simulink model "attitude_controllerV6"  (R2025a)
settings: Solver=FixedStepDiscrete  StartTime=0.0  StopTime=40  FixedStep=1e-4  RelTol=1e-6
undefined symbols (not defined in the file or in its folder): DiscIntNeverNeededParam
libraries: simulink x18, cstblocks x14, slpidlib x6, aerolibutil x2, rllib x1
(part 2 of 2)

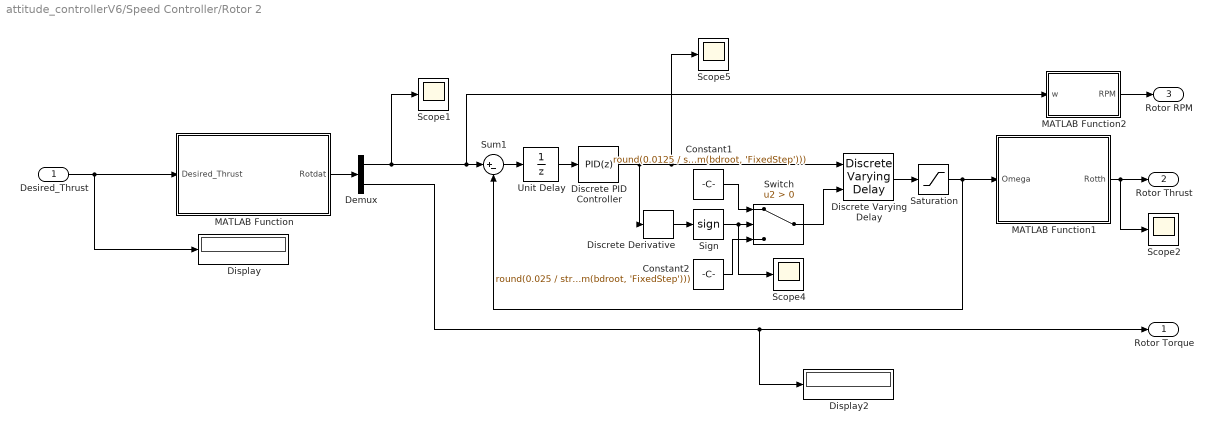
== system attitude_controllerV6/Speed Controller/Rotor 2 ==
  Desired_Thrust : Inport
  Constant1 : Constant  Value=round(0.0125 / str2double(get_param(bdroot, 'FixedStep')))
  Constant2 : Constant  Value=round(0.025 / str2double(get_param(bdroot, 'FixedStep')))
  Demux : Demux  Outputs=2
  Discrete Derivative : simulink/Discrete/Discrete Derivative  gainval=1.0  ICPrevScaledInput=0.0  OutMin=[]  OutMax=[]  OutDataType=fixdt(1, 16)  OutScaling=2^-10  DoSatur=off
  Discrete PID Controller : slpidlib/PID Controller  Controller=PID  Form=Parallel  TimeDomain=Discrete-time  UseExternalTs=off  SampleTime=-1  IntegratorMethod=Forward Euler  FilterMethod=Forward Euler  ControllerParametersSource=internal  P=0  I=30  UseKiTs=off  D=0  UseExternalDerivativeSource=off  N=100  UseFilter=on  TunerSelectOption=Transfer Function Based (PID Tuner App)  InitialConditionSource=internal  InitialConditionForIntegrator=0  InitialConditionForFilter=0  DifferentiatorICPrevScaledInput=0  ExternalReset=none  TrackingMode=off  Kt=1  LimitOutput=off  SatLimitsSource=internal  UpperSaturationLimit=inf  LowerSaturationLimit=-inf  LinearizeAsGain=off  AntiWindupMode=none  Kb=1  LimitIntegrator=off  UpperIntegratorSaturationLimit=inf  LowerIntegratorSaturationLimit=-inf  POutMin=[]  POutMax=[]  IOutMin=[]  IOutMax=[]  DOutMin=[]  DOutMax=[]  NOutMin=[]  NOutMax=[]  SumOutMin=[]  SumOutMax=[]  SaturationOutMin=[]  SaturationOutMax=[]  PParamMin=[]  PParamMax=[]  IParamMin=[]  IParamMax=[]  DParamMin=[]  DParamMax=[]  NParamMin=[]  NParamMax=[]  KbParamMin=[]  KbParamMax=[]  KtParamMin=[]  KtParamMax=[]  KbOutMin=[]  KbOutMax=[]  KtOutMin=[]  KtOutMax=[]  IntegratorOutMin=[]  IntegratorOutMax=[]  FilterOutMin=[]  FilterOutMax=[]  SumI1OutMin=[]  SumI1OutMax=[]  SumI2OutMin=[]  SumI2OutMax=[]  SumI3OutMin=[]  SumI3OutMax=[]  SumI4OutMin=[]  SumI4OutMax=[]  SumDOutMin=[]  SumDOutMax=[]  DifferentiatorOutMin=[]  DifferentiatorOutMax=[]  FilterDiffOutCoefMin=[]  FilterDiffOutCoefMax=[]  ReciprocalOutMin=[]  ReciprocalOutMax=[]  SumDenOutMin=[]  SumDenOutMax=[]  SumNumOutMin=[]  SumNumOutMax=[]  DivideOutMin=[]  DivideOutMax=[]  UdiffTsProdOutMin=[]  UdiffTsProdOutMax=[]  NTsProdOutMin=[]  NTsProdOutMax=[]  UintegralTsProdOutMin=[]  UintegralTsProdOutMax=[]  UngainTsProdOutMin=[]  UngainTsProdOutMax=[]  ClampingZeroOutDataTypeStr=Inherit: Inherit via back propagation  ClampingZeroOutMin=[]  ClampingZeroOutMax=[]  FilterDenConstantOutDataTypeStr=Inherit: Inherit via back propagation  FilterDenConstantOutMin=[]  FilterDenConstantOutMax=[]  PCopyOutDataTypeStr=Inherit: Inherit via back propagation  PCopyOutMin=[]  PCopyOutMax=[]  NCopyOutDataTypeStr=Inherit: Inherit via back propagation  NCopyOutMin=[]  NCopyOutMax=[]  IntegratorContinuousStateAttributes=''  IntegratorStateMustResolveToSignalObject=off  IntegratorRTWStateStorageClass=Auto  FilterContinuousStateAttributes=''  FilterStateMustResolveToSignalObject=off  FilterRTWStateStorageClass=Auto  ParallelPVariant=InternalParameters  IdealPVariant=Disabled  IVariant=InternalParameters  DVariant=InternalParameters  IntegratorVariant=Discrete  SatVariant=Disabled  AWVariant=Passthrough  PCopyVariant=Disabled  TRVariant=Disabled  FdbkBlocksVariant=Forward  IdealPFdbkVariant=Disabled  SatFdbkVariant=Disabled  DerivativeFilterVariant=ForwardEulerFilter  NVariant=InternalParameters  NCopyVariant=Disabled  FilterICVariant=InternalICsFilter  IntegratorICVariant=InternalICs  ExternalResetVariant=Disabled  TRSumVariant=Passthrough  SumFdbkVariant=Disabled  SumVariant=Sum_PID  TsampFilterVariant=InternalTs  TsampNgainVariant=Passthrough  TsampIntegralVariant=Disabled_SignalSpec  ExternalSaturationOutDataTypeStr=Inherit: Same as second input  DerivativeSourceVariant=ErrorSignal  PreIntVariant=InternalPreInt
      settings: LibrarySourceBlock=simulink/Discrete/Discrete PID Controller
  Discrete Varying Delay : cstblocks/Linear Parameter Varying/Discrete Varying Delay  Td=1  TdMax=10  TdFixed=[]  u0=0  Ts=-1  PreventDirectFeedthrough=off
  Display : Display
  Display2 : Display
  MATLAB Function : MATLAB Function  TreatAsAtomicUnit=on
  MATLAB Function1 : MATLAB Function  TreatAsAtomicUnit=on
  MATLAB Function2 : MATLAB Function  TreatAsAtomicUnit=on
  Saturation : Saturate  UpperLimit=1100  LowerLimit=0
  Scope{1..2,4..5} (4 alike) : Scope
      Scope1 settings: ActiveDisplayYMinimum=-154.8589621534594  ActiveDisplayYMaximum=1393.730659381135  DataLoggingVariableName=ScopeData4
      Scope2 settings: ActiveDisplayYMinimum=-0.6507136238694633  ActiveDisplayYMaximum=5.8564226148251706  DataLoggingVariableName=ScopeData5
      Scope4 settings: ActiveDisplayYMinimum=-1  ActiveDisplayYMaximum=1  DataLoggingVariableName=ScopeData12
      Scope5 settings: ActiveDisplayYMinimum=-115.66192536632313  ActiveDisplayYMaximum=1040.9573282969084  DataLoggingVariableName=ScopeData13
  Sign : Signum
  Sum1 : Sum  Inputs=|+-
  Switch : Switch  Criteria=u2 > Threshold  SaturateOnIntegerOverflow=off  InputSameDT=off
  Unit Delay : UnitDelay  SampleTime=-1  HasFrameUpgradeWarning=on
  Rotor Torque : Outport
  Rotor Thrust : Outport  Port=2
  Rotor RPM : Outport  Port=3
  wires:
  MATLAB Function2/1(RPM) -> Rotor RPM/1
  Sign/1 -> Switch/2, Scope4/1
  Discrete PID Controller/1 -> Discrete Derivative/1, Discrete Varying Delay/1, Scope5/1
  Constant1/1 -> Switch/1
  Discrete Derivative/1 -> Sign/1
  Discrete Varying Delay/1 -> Saturation/1
  Constant2/1 -> Switch/3
  Unit Delay/1 -> Discrete PID Controller/1
  Switch/1 -> Discrete Varying Delay/2
  Sum1/1 -> Unit Delay/1
  Saturation/1 -> Sum1/2, MATLAB Function1/1(Omega)
  Demux/2 -> Rotor Torque/1, Display2/1
  Desired_Thrust/1 -> MATLAB Function/1(Desired_Thrust), Display/1
  MATLAB Function/1(Rotdat) -> Demux/1
  MATLAB Function1/1(Rotth) -> Scope2/1, Rotor Thrust/1
  Demux/1 -> Scope1/1, Sum1/1, MATLAB Function2/1(w)

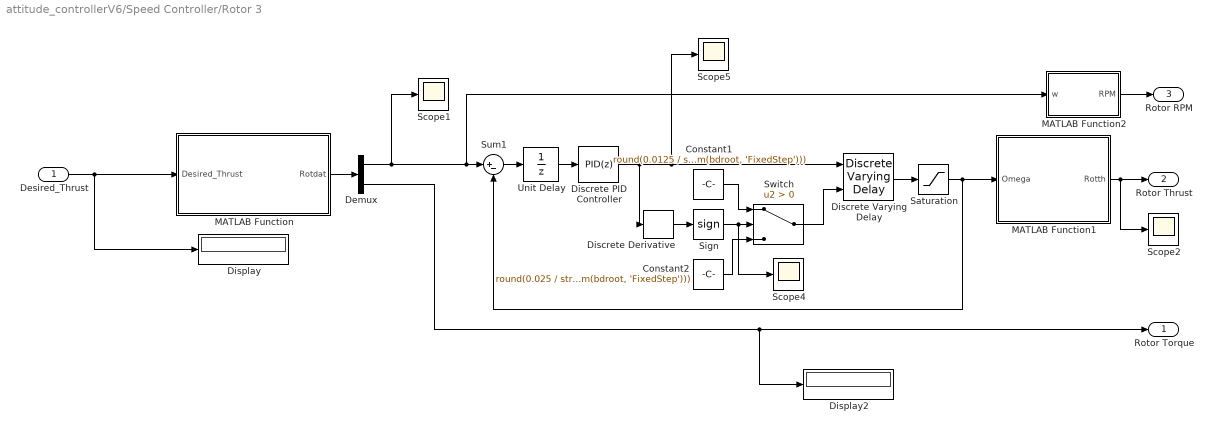
== system attitude_controllerV6/Speed Controller/Rotor 3 ==
  Desired_Thrust : Inport
  Constant1 : Constant  Value=round(0.0125 / str2double(get_param(bdroot, 'FixedStep')))
  Constant2 : Constant  Value=round(0.025 / str2double(get_param(bdroot, 'FixedStep')))
  Demux : Demux  Outputs=2
  Discrete Derivative : simulink/Discrete/Discrete Derivative  gainval=1.0  ICPrevScaledInput=0.0  OutMin=[]  OutMax=[]  OutDataType=fixdt(1, 16)  OutScaling=2^-10  DoSatur=off
  Discrete PID Controller : slpidlib/PID Controller  Controller=PID  Form=Parallel  TimeDomain=Discrete-time  UseExternalTs=off  SampleTime=-1  IntegratorMethod=Forward Euler  FilterMethod=Forward Euler  ControllerParametersSource=internal  P=0  I=30  UseKiTs=off  D=0  UseExternalDerivativeSource=off  N=100  UseFilter=on  TunerSelectOption=Transfer Function Based (PID Tuner App)  InitialConditionSource=internal  InitialConditionForIntegrator=0  InitialConditionForFilter=0  DifferentiatorICPrevScaledInput=0  ExternalReset=none  TrackingMode=off  Kt=1  LimitOutput=off  SatLimitsSource=internal  UpperSaturationLimit=inf  LowerSaturationLimit=-inf  LinearizeAsGain=off  AntiWindupMode=none  Kb=1  LimitIntegrator=off  UpperIntegratorSaturationLimit=inf  LowerIntegratorSaturationLimit=-inf  POutMin=[]  POutMax=[]  IOutMin=[]  IOutMax=[]  DOutMin=[]  DOutMax=[]  NOutMin=[]  NOutMax=[]  SumOutMin=[]  SumOutMax=[]  SaturationOutMin=[]  SaturationOutMax=[]  PParamMin=[]  PParamMax=[]  IParamMin=[]  IParamMax=[]  DParamMin=[]  DParamMax=[]  NParamMin=[]  NParamMax=[]  KbParamMin=[]  KbParamMax=[]  KtParamMin=[]  KtParamMax=[]  KbOutMin=[]  KbOutMax=[]  KtOutMin=[]  KtOutMax=[]  IntegratorOutMin=[]  IntegratorOutMax=[]  FilterOutMin=[]  FilterOutMax=[]  SumI1OutMin=[]  SumI1OutMax=[]  SumI2OutMin=[]  SumI2OutMax=[]  SumI3OutMin=[]  SumI3OutMax=[]  SumI4OutMin=[]  SumI4OutMax=[]  SumDOutMin=[]  SumDOutMax=[]  DifferentiatorOutMin=[]  DifferentiatorOutMax=[]  FilterDiffOutCoefMin=[]  FilterDiffOutCoefMax=[]  ReciprocalOutMin=[]  ReciprocalOutMax=[]  SumDenOutMin=[]  SumDenOutMax=[]  SumNumOutMin=[]  SumNumOutMax=[]  DivideOutMin=[]  DivideOutMax=[]  UdiffTsProdOutMin=[]  UdiffTsProdOutMax=[]  NTsProdOutMin=[]  NTsProdOutMax=[]  UintegralTsProdOutMin=[]  UintegralTsProdOutMax=[]  UngainTsProdOutMin=[]  UngainTsProdOutMax=[]  ClampingZeroOutDataTypeStr=Inherit: Inherit via back propagation  ClampingZeroOutMin=[]  ClampingZeroOutMax=[]  FilterDenConstantOutDataTypeStr=Inherit: Inherit via back propagation  FilterDenConstantOutMin=[]  FilterDenConstantOutMax=[]  PCopyOutDataTypeStr=Inherit: Inherit via back propagation  PCopyOutMin=[]  PCopyOutMax=[]  NCopyOutDataTypeStr=Inherit: Inherit via back propagation  NCopyOutMin=[]  NCopyOutMax=[]  IntegratorContinuousStateAttributes=''  IntegratorStateMustResolveToSignalObject=off  IntegratorRTWStateStorageClass=Auto  FilterContinuousStateAttributes=''  FilterStateMustResolveToSignalObject=off  FilterRTWStateStorageClass=Auto  ParallelPVariant=InternalParameters  IdealPVariant=Disabled  IVariant=InternalParameters  DVariant=InternalParameters  IntegratorVariant=Discrete  SatVariant=Disabled  AWVariant=Passthrough  PCopyVariant=Disabled  TRVariant=Disabled  FdbkBlocksVariant=Forward  IdealPFdbkVariant=Disabled  SatFdbkVariant=Disabled  DerivativeFilterVariant=ForwardEulerFilter  NVariant=InternalParameters  NCopyVariant=Disabled  FilterICVariant=InternalICsFilter  IntegratorICVariant=InternalICs  ExternalResetVariant=Disabled  TRSumVariant=Passthrough  SumFdbkVariant=Disabled  SumVariant=Sum_PID  TsampFilterVariant=InternalTs  TsampNgainVariant=Passthrough  TsampIntegralVariant=Disabled_SignalSpec  ExternalSaturationOutDataTypeStr=Inherit: Same as second input  DerivativeSourceVariant=ErrorSignal  PreIntVariant=InternalPreInt
      settings: LibrarySourceBlock=simulink/Discrete/Discrete PID Controller
  Discrete Varying Delay : cstblocks/Linear Parameter Varying/Discrete Varying Delay  Td=1  TdMax=10  TdFixed=[]  u0=0  Ts=-1  PreventDirectFeedthrough=off
  Display : Display
  Display2 : Display
  MATLAB Function : MATLAB Function  TreatAsAtomicUnit=on
  MATLAB Function1 : MATLAB Function  TreatAsAtomicUnit=on
  MATLAB Function2 : MATLAB Function  TreatAsAtomicUnit=on
  Saturation : Saturate  UpperLimit=1100  LowerLimit=0
  Scope{1..2,4..5} (4 alike) : Scope
      Scope1 settings: ActiveDisplayYMinimum=-154.8589621534594  ActiveDisplayYMaximum=1393.730659381135  DataLoggingVariableName=ScopeData4
      Scope2 settings: ActiveDisplayYMinimum=-0.6507136238694633  ActiveDisplayYMaximum=5.8564226148251706  DataLoggingVariableName=ScopeData5
      Scope4 settings: ActiveDisplayYMinimum=-1  ActiveDisplayYMaximum=1  DataLoggingVariableName=ScopeData12
      Scope5 settings: ActiveDisplayYMinimum=-115.66192536632313  ActiveDisplayYMaximum=1040.9573282969084  DataLoggingVariableName=ScopeData13
  Sign : Signum
  Sum1 : Sum  Inputs=|+-
  Switch : Switch  Criteria=u2 > Threshold  SaturateOnIntegerOverflow=off  InputSameDT=off
  Unit Delay : UnitDelay  SampleTime=-1  HasFrameUpgradeWarning=on
  Rotor Torque : Outport
  Rotor Thrust : Outport  Port=2
  Rotor RPM : Outport  Port=3
  wires:
  Demux/1 -> MATLAB Function2/1(w), Sum1/1, Scope1/1
  MATLAB Function1/1(Rotth) -> Rotor Thrust/1, Scope2/1
  MATLAB Function/1(Rotdat) -> Demux/1
  Desired_Thrust/1 -> Display/1, MATLAB Function/1(Desired_Thrust)
  Demux/2 -> Display2/1, Rotor Torque/1
  Saturation/1 -> MATLAB Function1/1(Omega), Sum1/2
  Sum1/1 -> Unit Delay/1
  Switch/1 -> Discrete Varying Delay/2
  Unit Delay/1 -> Discrete PID Controller/1
  Constant2/1 -> Switch/3
  Discrete Varying Delay/1 -> Saturation/1
  Discrete Derivative/1 -> Sign/1
  Constant1/1 -> Switch/1
  Discrete PID Controller/1 -> Scope5/1, Discrete Varying Delay/1, Discrete Derivative/1
  Sign/1 -> Scope4/1, Switch/2
  MATLAB Function2/1(RPM) -> Rotor RPM/1

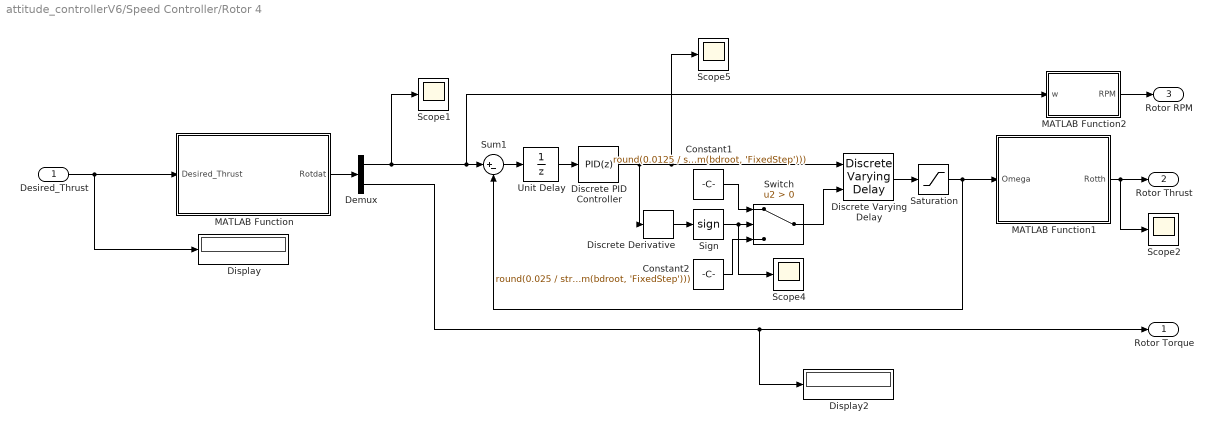
== system attitude_controllerV6/Speed Controller/Rotor 4 ==
  Desired_Thrust : Inport
  Constant1 : Constant  Value=round(0.0125 / str2double(get_param(bdroot, 'FixedStep')))
  Constant2 : Constant  Value=round(0.025 / str2double(get_param(bdroot, 'FixedStep')))
  Demux : Demux  Outputs=2
  Discrete Derivative : simulink/Discrete/Discrete Derivative  gainval=1.0  ICPrevScaledInput=0.0  OutMin=[]  OutMax=[]  OutDataType=fixdt(1, 16)  OutScaling=2^-10  DoSatur=off
  Discrete PID Controller : slpidlib/PID Controller  Controller=PID  Form=Parallel  TimeDomain=Discrete-time  UseExternalTs=off  SampleTime=-1  IntegratorMethod=Forward Euler  FilterMethod=Forward Euler  ControllerParametersSource=internal  P=0  I=30  UseKiTs=off  D=0  UseExternalDerivativeSource=off  N=100  UseFilter=on  TunerSelectOption=Transfer Function Based (PID Tuner App)  InitialConditionSource=internal  InitialConditionForIntegrator=0  InitialConditionForFilter=0  DifferentiatorICPrevScaledInput=0  ExternalReset=none  TrackingMode=off  Kt=1  LimitOutput=off  SatLimitsSource=internal  UpperSaturationLimit=inf  LowerSaturationLimit=-inf  LinearizeAsGain=off  AntiWindupMode=none  Kb=1  LimitIntegrator=off  UpperIntegratorSaturationLimit=inf  LowerIntegratorSaturationLimit=-inf  POutMin=[]  POutMax=[]  IOutMin=[]  IOutMax=[]  DOutMin=[]  DOutMax=[]  NOutMin=[]  NOutMax=[]  SumOutMin=[]  SumOutMax=[]  SaturationOutMin=[]  SaturationOutMax=[]  PParamMin=[]  PParamMax=[]  IParamMin=[]  IParamMax=[]  DParamMin=[]  DParamMax=[]  NParamMin=[]  NParamMax=[]  KbParamMin=[]  KbParamMax=[]  KtParamMin=[]  KtParamMax=[]  KbOutMin=[]  KbOutMax=[]  KtOutMin=[]  KtOutMax=[]  IntegratorOutMin=[]  IntegratorOutMax=[]  FilterOutMin=[]  FilterOutMax=[]  SumI1OutMin=[]  SumI1OutMax=[]  SumI2OutMin=[]  SumI2OutMax=[]  SumI3OutMin=[]  SumI3OutMax=[]  SumI4OutMin=[]  SumI4OutMax=[]  SumDOutMin=[]  SumDOutMax=[]  DifferentiatorOutMin=[]  DifferentiatorOutMax=[]  FilterDiffOutCoefMin=[]  FilterDiffOutCoefMax=[]  ReciprocalOutMin=[]  ReciprocalOutMax=[]  SumDenOutMin=[]  SumDenOutMax=[]  SumNumOutMin=[]  SumNumOutMax=[]  DivideOutMin=[]  DivideOutMax=[]  UdiffTsProdOutMin=[]  UdiffTsProdOutMax=[]  NTsProdOutMin=[]  NTsProdOutMax=[]  UintegralTsProdOutMin=[]  UintegralTsProdOutMax=[]  UngainTsProdOutMin=[]  UngainTsProdOutMax=[]  ClampingZeroOutDataTypeStr=Inherit: Inherit via back propagation  ClampingZeroOutMin=[]  ClampingZeroOutMax=[]  FilterDenConstantOutDataTypeStr=Inherit: Inherit via back propagation  FilterDenConstantOutMin=[]  FilterDenConstantOutMax=[]  PCopyOutDataTypeStr=Inherit: Inherit via back propagation  PCopyOutMin=[]  PCopyOutMax=[]  NCopyOutDataTypeStr=Inherit: Inherit via back propagation  NCopyOutMin=[]  NCopyOutMax=[]  IntegratorContinuousStateAttributes=''  IntegratorStateMustResolveToSignalObject=off  IntegratorRTWStateStorageClass=Auto  FilterContinuousStateAttributes=''  FilterStateMustResolveToSignalObject=off  FilterRTWStateStorageClass=Auto  ParallelPVariant=InternalParameters  IdealPVariant=Disabled  IVariant=InternalParameters  DVariant=InternalParameters  IntegratorVariant=Discrete  SatVariant=Disabled  AWVariant=Passthrough  PCopyVariant=Disabled  TRVariant=Disabled  FdbkBlocksVariant=Forward  IdealPFdbkVariant=Disabled  SatFdbkVariant=Disabled  DerivativeFilterVariant=ForwardEulerFilter  NVariant=InternalParameters  NCopyVariant=Disabled  FilterICVariant=InternalICsFilter  IntegratorICVariant=InternalICs  ExternalResetVariant=Disabled  TRSumVariant=Passthrough  SumFdbkVariant=Disabled  SumVariant=Sum_PID  TsampFilterVariant=InternalTs  TsampNgainVariant=Passthrough  TsampIntegralVariant=Disabled_SignalSpec  ExternalSaturationOutDataTypeStr=Inherit: Same as second input  DerivativeSourceVariant=ErrorSignal  PreIntVariant=InternalPreInt
      settings: LibrarySourceBlock=simulink/Discrete/Discrete PID Controller
  Discrete Varying Delay : cstblocks/Linear Parameter Varying/Discrete Varying Delay  Td=1  TdMax=10  TdFixed=[]  u0=0  Ts=-1  PreventDirectFeedthrough=off
  Display : Display
  Display2 : Display
  MATLAB Function : MATLAB Function  TreatAsAtomicUnit=on
  MATLAB Function1 : MATLAB Function  TreatAsAtomicUnit=on
  MATLAB Function2 : MATLAB Function  TreatAsAtomicUnit=on
  Saturation : Saturate  UpperLimit=1100  LowerLimit=0
  Scope{1..2,4..5} (4 alike) : Scope
      Scope1 settings: ActiveDisplayYMinimum=-154.8589621534594  ActiveDisplayYMaximum=1393.730659381135  DataLoggingVariableName=ScopeData4
      Scope2 settings: ActiveDisplayYMinimum=-0.6507136238694633  ActiveDisplayYMaximum=5.8564226148251706  DataLoggingVariableName=ScopeData5
      Scope4 settings: ActiveDisplayYMinimum=-1  ActiveDisplayYMaximum=1  DataLoggingVariableName=ScopeData12
      Scope5 settings: ActiveDisplayYMinimum=-115.66192536632313  ActiveDisplayYMaximum=1040.9573282969084  DataLoggingVariableName=ScopeData13
  Sign : Signum
  Sum1 : Sum  Inputs=|+-
  Switch : Switch  Criteria=u2 > Threshold  SaturateOnIntegerOverflow=off  InputSameDT=off
  Unit Delay : UnitDelay  SampleTime=-1  HasFrameUpgradeWarning=on
  Rotor Torque : Outport
  Rotor Thrust : Outport  Port=2
  Rotor RPM : Outport  Port=3
  wires:
  MATLAB Function2/1(RPM) -> Rotor RPM/1
  Sign/1 -> Switch/2, Scope4/1
  Discrete PID Controller/1 -> Discrete Derivative/1, Discrete Varying Delay/1, Scope5/1
  Constant1/1 -> Switch/1
  Discrete Derivative/1 -> Sign/1
  Discrete Varying Delay/1 -> Saturation/1
  Constant2/1 -> Switch/3
  Unit Delay/1 -> Discrete PID Controller/1
  Switch/1 -> Discrete Varying Delay/2
  Sum1/1 -> Unit Delay/1
  Saturation/1 -> Sum1/2, MATLAB Function1/1(Omega)
  Demux/2 -> Rotor Torque/1, Display2/1
  Desired_Thrust/1 -> MATLAB Function/1(Desired_Thrust), Display/1
  MATLAB Function/1(Rotdat) -> Demux/1
  MATLAB Function1/1(Rotth) -> Scope2/1, Rotor Thrust/1
  Demux/1 -> Scope1/1, Sum1/1, MATLAB Function2/1(w)

== system attitude_controllerV6/Gyro/noise/Subsystem1 ==
  "  " : Inport
  Selector : Selector  InputPortWidth=3  IndexOptions=Index vector (dialog)  Indices=[1]  OutputSizes=1
  Selector1 : Selector  InputPortWidth=3  IndexOptions=Index vector (dialog)  Indices=[2]  OutputSizes=1
  Selector2 : Selector  InputPortWidth=3  IndexOptions=Index vector (dialog)  Indices=[3]  OutputSizes=1
  Out1 : Outport
  Out2 : Outport  Port=2
  Out3 : Outport  Port=3
  wires:
  Selector2/1 -> Out3/1
  Selector1/1 -> Out2/1
  Selector/1 -> Out1/1
  "  "/1 -> Selector2/1, Selector/1, Selector1/1

== system attitude_controllerV6/Position Control/Subsystem3/Subsystem1 ==
  u : Inport
  Abs1 : Abs  SaturateOnIntegerOverflow=off
  MATLAB Function : MATLAB Function  TreatAsAtomicUnit=on
  Scope : Scope
      settings: ActiveDisplayYMinimum=-1  ActiveDisplayYMaximum=1  DataLoggingVariableName=ScopeData2
  Scope1 : Scope
      settings: ActiveDisplayYMinimum=-0.21788976949861752  ActiveDisplayYMaximum=1.1353210854998463  DataLoggingVariableName=ScopeData14
  y : Outport
  wires:
  MATLAB Function/1(y) -> Scope/1, y/1
  u/1 -> Abs1/1
  Abs1/1 -> Scope1/1, MATLAB Function/1(u)

== system attitude_controllerV6/Position Control/Subsystem3/Subsystem5 ==
  u : Inport
  Abs1 : Abs  SaturateOnIntegerOverflow=off
  MATLAB Function : MATLAB Function  TreatAsAtomicUnit=on
  Scope : Scope
      settings: ActiveDisplayYMinimum=7.125  ActiveDisplayYMaximum=15.875  DataLoggingVariableName=ScopeData2
  Scope1 : Scope
      settings: ActiveDisplayYMinimum=-0.21788976949861752  ActiveDisplayYMaximum=1.1353210854998463  DataLoggingVariableName=ScopeData14
  y : Outport
  wires:
  MATLAB Function/1(y) -> y/1, Scope/1
  u/1 -> Abs1/1
  Abs1/1 -> MATLAB Function/1(u), Scope1/1

== system attitude_controllerV6/Position Control/Subsystem4/Subsystem1 ==
  u : Inport
  Abs1 : Abs  SaturateOnIntegerOverflow=off
  MATLAB Function : MATLAB Function  TreatAsAtomicUnit=on
  Scope : Scope
      settings: ActiveDisplayYMinimum=-1  ActiveDisplayYMaximum=1  DataLoggingVariableName=ScopeData2
  Scope1 : Scope
      settings: ActiveDisplayYMinimum=-0.21788976949861752  ActiveDisplayYMaximum=1.1353210854998463  DataLoggingVariableName=ScopeData14
  y : Outport
  wires:
  MATLAB Function/1(y) -> y/1, Scope/1
  u/1 -> Abs1/1
  Abs1/1 -> MATLAB Function/1(u), Scope1/1

== system attitude_controllerV6/Position Control/Subsystem4/Subsystem5 ==
  u : Inport
  Abs1 : Abs  SaturateOnIntegerOverflow=off
  MATLAB Function : MATLAB Function  TreatAsAtomicUnit=on
  Scope : Scope
      settings: ActiveDisplayYMinimum=7.125  ActiveDisplayYMaximum=15.875  DataLoggingVariableName=ScopeData2
  Scope1 : Scope
      settings: ActiveDisplayYMinimum=-0.21788976949861752  ActiveDisplayYMaximum=1.1353210854998463  DataLoggingVariableName=ScopeData14
  y : Outport
  wires:
  u/1 -> Abs1/1
  MATLAB Function/1(y) -> Scope/1, y/1
  Abs1/1 -> Scope1/1, MATLAB Function/1(u)

== matlab function attitude_controllerV6/Attitude Control/Quaternion P control/MATLAB Function1 ==
  data: eul input; quat output
function quat = eulTOquat(eul)
eulv = [eul(1) eul(2) eul(3)];
quatr = eul2quat(eulv, 'XYZ');
quat = quatr(:);
end

== matlab function attitude_controllerV6/Speed Controller/Rotor 4/MATLAB Function ==
  data: Desired_Thrust input; Rotdat output
function Rotdat = ThrustToOmegaTau(Desired_Thrust)
Kt = 5.84e-06; % Kt rotor thrust constant
Cm = 0.06;     % Kq rotor torque constant


if Desired_Thrust >= 0
    omega = sqrt((Desired_Thrust/Kt));
else
    omega = 0;
end


%omega = sqrt((Desired_Thrust/Kt));
torque = Kt*Cm*(omega^2);

Rotdat = [omega; torque];
end

== matlab function attitude_controllerV6/Speed Controller/Rotor 4/MATLAB Function1 ==
  data: Omega input; Rotth output
function Rotth = RotorThrust(Omega)
Kt = 5.84e-06; % Kt rotor thrust constant

Rotth = Kt*(Omega^2);
end

== matlab function attitude_controllerV6/Speed Controller/Rotor 4/MATLAB Function2 ==
  data: w input; RPM output
function RPM = WtoRPM(w)

RPM = (w*60)/(2*pi);

== matlab function attitude_controllerV6/Speed Controller/MATLAB Function ==
  data: r1t input; torth output; r1th input; r2t input; r2th input; r3t input; r3th input; r4t input; r4th input
function torth = Torque_Experienced(r1t,r1th,r2t,r2th,r3t,r3th,r4t,r4th)
mtm = 0.55; % Motor to motor distance - m
rt = [r1t; -r2t; -r3t; r4t]; % rotor torques
Xtor = ((r1th*mtm)+(r2th*mtm)) - ((r3th*mtm)+(r4th*mtm));     % x axis torque (pitch up is +)
Ytor = ((r1th*mtm)+(r3th*mtm)) - ((r2th*mtm)+(r4th*mtm));     % y axis torque (roll right is +)
Ztor = sum(rt, "all"); % z axis torque (yaw left is +)
thrusttot = r1th+r2th+r3th+r4th; % total thrust
torth = [Xtor; Ytor; Ztor; thrusttot]; % Torque matrix
end

== matlab function attitude_controllerV6/Speed Controller/Rotor 1/MATLAB Function ==
  data: Desired_Thrust input; Rotdat output
function Rotdat = ThrustToOmegaTau(Desired_Thrust)
Kt = 5.84e-06; % Kt rotor thrust constant
Cm = 0.06;     % Kq rotor torque constant


if Desired_Thrust >= 0
    omega = sqrt((Desired_Thrust/Kt));
else
    omega = 0;
end


%omega = sqrt((Desired_Thrust/Kt));
torque = Kt*Cm*(omega^2);

Rotdat = [omega; torque];
end

== matlab function attitude_controllerV6/Speed Controller/Rotor 1/MATLAB Function1 ==
  data: Omega input; Rotth output
function Rotth = RotorThrust(Omega)
Kt = 5.84e-06; % Kt rotor thrust constant

Rotth = Kt*(Omega^2);
end

== matlab function attitude_controllerV6/Position Control/Subsystem3/Subsystem5/MATLAB Function ==
  data: u input; y output
function y = fcn(u)
a = 0;
if u < 0.4
    a = 15;
end
if u <= 1 && u >= 0.4
    a = 8*(u^-0.686);
end
if u > 1
    a = 8;
end

y = a;

== matlab function attitude_controllerV6/Position Control/Subsystem3/Subsystem1/MATLAB Function ==
  data: u input; y output
function y = fcn(u)
a = 0;
if u < 0.4
    a = 6;
end
if u <= 15 && u >= 0.4
    a = 5.3592*(u^-0.094);
end
if u > 15
    a = 4;
end

y = a;

== matlab function attitude_controllerV6/Dynamic Model/MATLAB Function1 ==
  data: a output; torque input; thrust input; qdlin input; qdang input; qang input; wind input
function a = dynamics(torque, thrust, qdlin, qdang, qang, wind)
% torth = [Xtor; Ytor; Ztor; thrusttot];
%% Drone Parameters
MassD = 1.282; % Mass of Drone - Kg
g = 9.81; % Acceleration due to gravity - m/s^2
gref = [0; 0; -g]; % gravity in reference frame
rho = 1.225; % air density amsl kgm-3

etad = [qang(1); qang(2); qang(3)]; % rotation
eta = [deg2rad(etad(1)); deg2rad(etad(2)); deg2rad(etad(3))]; % rotation
vel = [qdlin(1); qdlin(2); qdlin(3)]; % uav velocity ms-1
RelWin = -vel+wind; % relative airspeed caused by movement through air
Fi = [0;0;thrust]; % Thrust
%% Rotation matrix
Rgx = [1 0      0;
      0 cos(eta(1))  sin(eta(1));
      0 -sin(eta(1)) cos(eta(1))];
Rgy = [cos(eta(2)) 0 sin(eta(2));
      0           1 0;
      -sin(eta(2)) 0 cos(eta(2))];
Rgz = [cos(eta(3)) -sin(eta(3)) 0;
      sin(eta(3)) cos(eta(3))  0;
      0           0            1];
RotBtR = Rgz*Rgy*Rgx; % body to reference frame rotation
%% inertia matrix
ixx = 0.029125;
iyy = 0.029125;
izz = 0.055225;
I = diag([ixx, iyy, izz]);
%% Gravity force matrix
Fg = (RotBtR'*gref); % gravitational acceleration (xyz) in body frame
Fgf = Fg*MassD; % gravitational force (xyz) in body frame
%% Drag force
%linear
cdyi = 0.1150546; % cd at 0ms-1
cdm = 5.8454e-3; % cd multiplier (gradient for cd/speed)
Cdlin = [cdyi+(cdm*qdlin(1));cdyi+(cdm*qdlin(2)) ;cdyi+(cdm*qdlin(3)) ]; % Coefficient of drage estimate
WArea = [0.017; 0.014; 0.047]; % Wind facing area estimate m^2 - from 3d model (y is front)
Fd = [0.5*rho*Cdlin(1)*WArea(1)*RelWin(1); 0.5*rho*Cdlin(2)*WArea(2)*RelWin(2); 0.5*rho*Cdlin(3)*WArea(3)*RelWin(3)]; % Drag Force matrix
%rotation
Cdrot = [cdyi+(cdm*qdang(1));cdyi+(cdm*qdang(2)) ;cdyi+(cdm*qdang(3)) ];
RArea = [0.047;0.047;0.012];
Cti = [0.5*rho*RArea(1)*Cdrot(1);0.5*rho*RArea(2)*Cdrot(2);0.5*rho*RArea(3)*Cdrot(3)];
Taudr = [(qdang(1)^2)*Cti(1); (qdang(2)^2)*Cti(2); (qdang(3)^2)*Cti(3)];
if qdang(1) > 0 
    Taudr(1) = -Taudr(1);
else
    Taudr(1) = Taudr(1);
end
if qdang(2) > 0
    Taudr(2) = -Taudr(2);
else
    Taudr(2) = Taudr(2);
end
if qdang(3) > 0
    Taudr(3) = -Taudr(3);
else
    Taudr(3) = Taudr(3);
end
%% acceleration
% linear acceleration
abx = (Fgf(1)+Fd(1))/MassD; % body x axis acceleration
aby = (Fgf(2)+Fd(2))/MassD; % body y axis acceleration
abz = (Fi(3) + Fgf(3) + Fd(3))/MassD; % body z axis acceleration
alinb = [abx; aby; abz];
alinr = RotBtR*alinb; % body to reference frame conversion
alin = [alinb(1); alinb(2); alinb(3); alinr(1); alinr(2); alinr(3);]; % linear acceleration - [body frame ; ref frame]
% angular acceleration
tau = [torque(1)+Taudr(1); torque(2)+Taudr(2); torque(3)+Taudr(3)];
vrotb = [qdang(1); qdang(2); qdang(3)];

arotb = I \ (tau - cross(vrotb, I*vrotb)); %[ixx*tau(1);iyy*tau(2);izz*tau(3)]; 
arotr = RotBtR*arotb;
arot = [arotb(1); arotb(2); arotb(3); arotr(1); arotr(2); arotr(3);]; %rotational acceleration

a = [alin; arot];

end

== matlab function attitude_controllerV6/Position Control/Subsystem4/Subsystem1/MATLAB Function ==
  data: u input; y output
function y = fcn(u)
a = 0;
if u < 0.4
    a = 6;
end
if u <= 15 && u >= 0.4
    a = 5.3592*(u^-0.094);
end
if u > 15
    a = 4;
end

y = a;

== matlab function attitude_controllerV6/Position Control/Subsystem4/Subsystem5/MATLAB Function ==
  data: u input; y output
function y = fcn(u)
a = 0;
if u < 0.4
    a = 15;
end
if u <= 1 && u >= 0.4
    a = 8*(u^-0.686);
end
if u > 1
    a = 8;
end

y = a;

== matlab function attitude_controllerV6/Position Control/Subsystem5/MATLAB Function ==
  data: u input; y output
function y = fcn(u)
a = 0;
if u <= 0.4
    a = 0.5;
end
if u > 0.4
    a = 0.3392*(u^-0.317);
end

y = a;

== matlab function attitude_controllerV6/Speed Controller/Rotor 2/MATLAB Function ==
  data: Desired_Thrust input; Rotdat output
function Rotdat = ThrustToOmegaTau(Desired_Thrust)
Kt = 5.84e-06; % Kt rotor thrust constant
Cm = 0.06;     % Kq rotor torque constant


if Desired_Thrust >= 0
    omega = sqrt((Desired_Thrust/Kt));
else
    omega = 0;
end


%omega = sqrt((Desired_Thrust/Kt));
torque = Kt*Cm*(omega^2);

Rotdat = [omega; torque];
end

== matlab function attitude_controllerV6/Speed Controller/Rotor 2/MATLAB Function1 ==
  data: Omega input; Rotth output
function Rotth = RotorThrust(Omega)
Kt = 5.84e-06; % Kt rotor thrust constant

Rotth = Kt*(Omega^2);
end

== matlab function attitude_controllerV6/Speed Controller/Rotor 2/MATLAB Function2 ==
  data: w input; RPM output
function RPM = WtoRPM(w)

RPM = (w*60)/(2*pi);

== matlab function attitude_controllerV6/Speed Controller/Rotor 3/MATLAB Function ==
  data: Desired_Thrust input; Rotdat output
function Rotdat = ThrustToOmegaTau(Desired_Thrust)
Kt = 5.84e-06; % Kt rotor thrust constant
Cm = 0.06;     % Kq rotor torque constant


if Desired_Thrust >= 0
    omega = sqrt((Desired_Thrust/Kt));
else
    omega = 0;
end


%omega = sqrt((Desired_Thrust/Kt));
torque = Kt*Cm*(omega^2);

Rotdat = [omega; torque];
end

== matlab function attitude_controllerV6/Speed Controller/Rotor 3/MATLAB Function1 ==
  data: Omega input; Rotth output
function Rotth = RotorThrust(Omega)
Kt = 5.84e-06; % Kt rotor thrust constant

Rotth = Kt*(Omega^2);
end

== matlab function attitude_controllerV6/Mixer ==
  data: alt input; DesTh output; Xrot input; Yrot input; Zrot input
function DesTh = mixer(alt, Xrot, Yrot, Zrot)

M1 = alt/4 - Xrot/2 - Yrot/2 - Zrot/4;
M2 = alt/4 - Xrot/2 + Yrot/2 + Zrot/4;
M3 = alt/4 + Xrot/2 - Yrot/2 + Zrot/4;
M4 = alt/4 + Xrot/2 + Yrot/2 - Zrot/4;

DesTh = [M1; M2; M3; M4];

== matlab function attitude_controllerV6/Speed Controller/Rotor 3/MATLAB Function2 ==
  data: w input; RPM output
function RPM = WtoRPM(w)

RPM = (w*60)/(2*pi);

== matlab function attitude_controllerV6/Position Control/Subsystem6/MATLAB Function ==
  data: u input; y output
function y = fcn(u)
a = 0;
if u <= 0.4
    a = 0.5;
end
if u > 0.4
    a = 0.3392*(u^-0.317);
end

y = a;

== matlab function attitude_controllerV6/Speed Controller/Rotor 1/MATLAB Function2 ==
  data: w input; RPM output
function RPM = WtoRPM(w)

RPM = (w*60)/(2*pi);

== matlab function attitude_controllerV6/Attitude Control/Quaternion P control/MATLAB Function ==
  data: eul input; quat output
function quat = eulTOquat(eul)
eulv = [eul(1) eul(2) eul(3)];
quatr = eul2quat(eulv, 'XYZ');
quat = quatr(:);
end
